simulink model "model"  (R2020b)
settings: Solver=VariableStepAuto  StartTime=0.0  StopTime=10.0  RelTol=1e-3
settings Model: Creator=SAGAR  LastModifiedBy=SAGAR

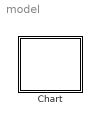
== system model ==
  Chart : Stateflow chart  TreatAsAtomicUnit=on

== stateflow chart model/Chart ==
  state stop
    y1=red;
    y2=green;
  state stopfortraffic
    y1=red;
    y2=green;
  state stoptogo
    y1=red;
    y2=yellow;
  state gotostop
    y1=yellow;
    y2=red;
  state go
    y1=green;
    y2=red;
  (default) -> stop
  stop -> stopfortraffic : after(20,tick)
  stopfortraffic -> stoptogo : [sens]
  gotostop -> stop : after(3,tick)
  stoptogo -> go : after(3,tick)
  go -> gotostop : after(10,tick)
